simulink model "homework2_discrete"  (R2018b)
settings: Solver=VariableStepAuto  StartTime=0.0  StopTime=10.0  RelTol=1e-3
values from neighbouring files (symbols this model uses):
  b = 100    [homework2.m]
  m = 1000    [homework2.m]
settings Model: Creator=Henkka  LastModifiedBy=Henkka

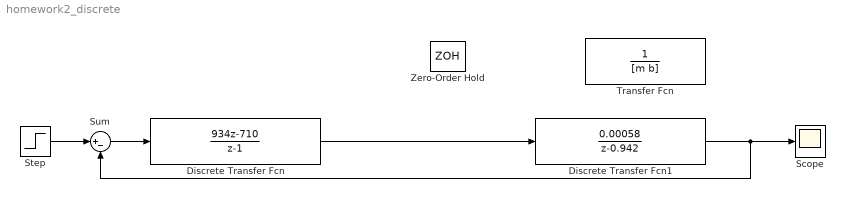
== system homework2_discrete ==
  Discrete Transfer Fcn : DiscreteTransferFcn  Numerator=[934 -710]  Denominator=[1 -1]
  Discrete Transfer Fcn1 : DiscreteTransferFcn  Numerator=[0.00058]  Denominator=[1 -0.942]
  Scope : Scope
  Step : Step  Time=0  After=100  SampleTime=0
  Sum : Sum  Inputs=|+-
  Transfer Fcn : TransferFcn  Denominator=[m b]
  Zero-Order Hold : ZeroOrderHold  SampleTime=-1
  wires:
  Sum/1 -> Discrete Transfer Fcn/1
  Step/1 -> Sum/1
  Discrete Transfer Fcn1/1 -> Sum/2, Scope/1
  Discrete Transfer Fcn/1 -> Discrete Transfer Fcn1/1
